simulink model "PreBrakingModel"  (Simulink 8.0)
settings: Solver=ode5  SolverMode=SingleTasking  StartTime=0.0  StopTime=inf  FixedStep=1/1000  RelTol=1e-3
libraries: simulink x27, simulink_extras x2
(part 2 of 2)

== system PreBrakingModel/PreBraking Model/Display module/Display ==
  RPM : Inport
  V : Inport  Port=2
  BrakePressure : Inport  Port=3
  Throttle : Inport  Port=4
  Warning flag 2.6s : Inport  Port=5
  Enable : EnablePort  PropagateVarSize=During execution
  Brake Pressure [bar] : Gain  Gain=100/MaxBrakePressure
  DISPLAY : M-S-Function  FunctionName=msfcn_AEBS_PlotSpeed  Parameters=DisplayFreq DisplaySwitch
  Logical Operator1 : Logic  Operator=OR  Inputs=1  AllPortsSameDT=off  OutDataTypeStr=boolean
  Rounding Function{,1..3} (4 alike) : Rounding  Operator=round  SampleTime=1/DisplayFreq
  wires:
  Rounding Function/1 -> DISPLAY/1
  Rounding Function1/1 -> DISPLAY/2
  Rounding Function2/1 -> DISPLAY/3
  Rounding Function3/1 -> DISPLAY/4
  Brake Pressure [bar]/1 -> Rounding Function2/1
  Logical Operator1/1 -> DISPLAY/5
  RPM/1 -> Rounding Function/1
  V/1 -> Rounding Function1/1
  BrakePressure/1 -> Brake Pressure [bar]/1
  Throttle/1 -> Rounding Function3/1
  Warning flag 2.6s/1 -> Logical Operator1/1

== system PreBrakingModel/PreBraking Model/Interpretation/If Action Subsystem ==
  Action Port : ActionPort  PropagateVarSize=During execution  ActionType=then
  Constant : Constant
  Data Store Write : DataStoreWrite  DataStoreName=full
  wires:
  Constant/1 -> Data Store Write/1

== system PreBrakingModel/PreBraking Model/Interpretation/If Action Subsystem1 ==
  Action Port : ActionPort  PropagateVarSize=During execution  ActionType=then
  Constant : Constant
  Data Store Write : DataStoreWrite  DataStoreName=part
  wires:
  Constant/1 -> Data Store Write/1

== system PreBrakingModel/PreBraking Model/Interpretation/If Action Subsystem2 ==
  Action Port : ActionPort  PropagateVarSize=During execution  ActionType=then
  Constant : Constant  Value=0  SampleTime=min(Tsensor)
  Data Store Write : DataStoreWrite  DataStoreName=part
  wires:
  Constant/1 -> Data Store Write/1

== system PreBrakingModel/PreBraking Model/Radar/Radar ==
  TIS1 Range : Inport
  TIS1 Theta : Inport  Port=2
  TIS2 Range : Inport  Port=3
  TIS2 Theta : Inport  Port=4
  all_flags1.6 : Inport  Port=5
  all_flags2.6 : Inport  Port=6
  all_flags0.6 : Inport  Port=7
  Enable : EnablePort  PropagateVarSize=During execution
  Level-2 M-file S-Function : M-S-Function  FunctionName=msfcn_AEBS_radar_graph  Parameters=RadarFreq TISdet TISMaxRange TISMaxTheta RadarSwitch
  wires:
  TIS1 Range/1 -> Level-2 M-file S-Function/1
  TIS1 Theta/1 -> Level-2 M-file S-Function/2
  TIS2 Range/1 -> Level-2 M-file S-Function/3
  TIS2 Theta/1 -> Level-2 M-file S-Function/4
  all_flags1.6/1 -> Level-2 M-file S-Function/5
  all_flags2.6/1 -> Level-2 M-file S-Function/6
  all_flags0.6/1 -> Level-2 M-file S-Function/7

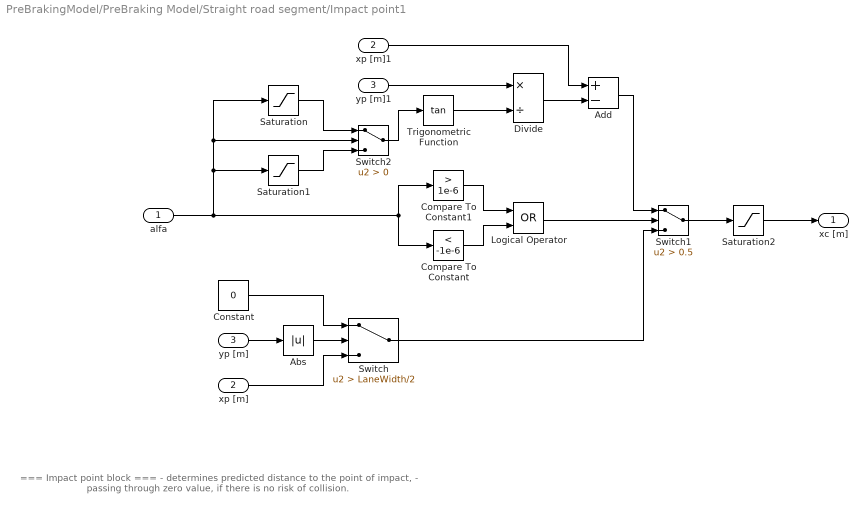
== system PreBrakingModel/PreBraking Model/Straight road segment/Impact point1 ==
  note: === Impact point block ===
      |
      |    - determines predicted distance to the point of impact,
      |    - passing through zero value, if there is no risk of collision.
  alfa : Inport
  xp [m] : Inport  Port=2
  yp [m] : Inport  Port=3
  Abs : Abs
  Add : Sum  Inputs=+-
  Compare To Constant : simulink/Logic and Bit Operations/Compare To Constant  relop=<  const=-1e-6  OutDataTypeStr=uint8  ZeroCross=off
  Compare To Constant1 : simulink/Logic and Bit Operations/Compare To Constant  relop=>  const=1e-6  OutDataTypeStr=uint8  ZeroCross=off
  Constant : Constant  Value=0
  Divide : Product  Inputs=*/
  Logical Operator : Logic  Operator=OR  AllPortsSameDT=off  OutDataTypeStr=boolean
  Saturation : Saturate  UpperLimit=inf  LowerLimit=1e-6
  Saturation1 : Saturate  UpperLimit=-1e-6  LowerLimit=-inf
  Saturation2 : Saturate  UpperLimit=300  LowerLimit=0
  Switch : Switch  Criteria=u2 > Threshold  Threshold=LaneWidth/2
  Switch1 : Switch  Criteria=u2 > Threshold  Threshold=0.5
  Switch2 : Switch  Criteria=u2 > Threshold
  Trigonometric Function : Trigonometry  Operator=tan
  xp [m]1 : InportShadow  Port=2
  yp [m]1 : InportShadow  Port=3
  xc [m] : Outport
  wires:
  yp [m]/1 -> Abs/1
  xp [m]/1 -> Switch/3
  Constant/1 -> Switch/1
  Switch/1 -> Switch1/3
  Abs/1 -> Switch/2
  xp [m]1/1 -> Add/1
  Divide/1 -> Add/2
  yp [m]1/1 -> Divide/1
  Trigonometric Function/1 -> Divide/2
  alfa/1 -> Compare To Constant1/1, Compare To Constant/1, Saturation1/1, Switch2/2, Saturation/1
  Compare To Constant1/1 -> Logical Operator/1
  Compare To Constant/1 -> Logical Operator/2
  Logical Operator/1 -> Switch1/2
  Switch1/1 -> Saturation2/1
  Add/1 -> Switch1/1
  Switch2/1 -> Trigonometric Function/1
  Saturation/1 -> Switch2/1
  Saturation1/1 -> Switch2/3
  Saturation2/1 -> xc [m]/1

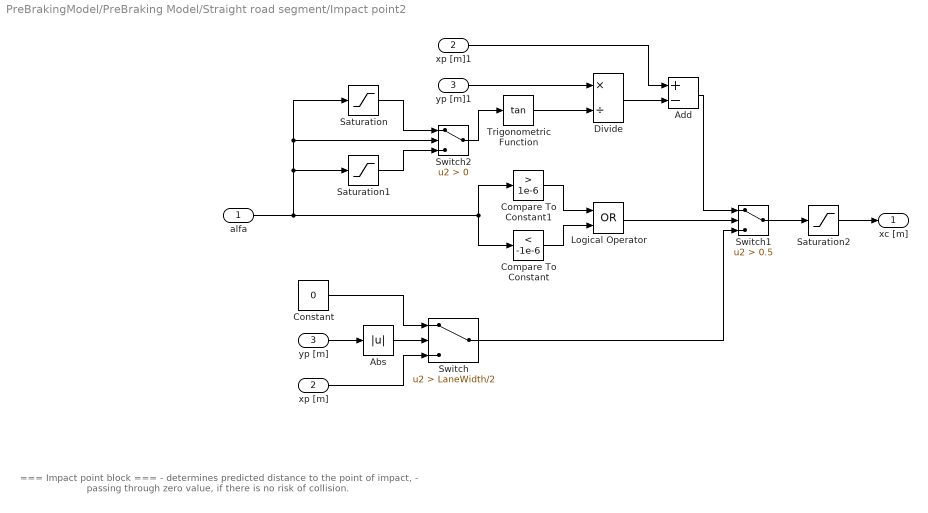
== system PreBrakingModel/PreBraking Model/Straight road segment/Impact point2 ==
  note: === Impact point block ===
      |
      |    - determines predicted distance to the point of impact,
      |    - passing through zero value, if there is no risk of collision.
  alfa : Inport
  xp [m] : Inport  Port=2
  yp [m] : Inport  Port=3
  Abs : Abs
  Add : Sum  Inputs=+-
  Compare To Constant : simulink/Logic and Bit Operations/Compare To Constant  relop=<  const=-1e-6  OutDataTypeStr=uint8  ZeroCross=off
  Compare To Constant1 : simulink/Logic and Bit Operations/Compare To Constant  relop=>  const=1e-6  OutDataTypeStr=uint8  ZeroCross=off
  Constant : Constant  Value=0
  Divide : Product  Inputs=*/
  Logical Operator : Logic  Operator=OR  AllPortsSameDT=off  OutDataTypeStr=boolean
  Saturation : Saturate  UpperLimit=inf  LowerLimit=1e-6
  Saturation1 : Saturate  UpperLimit=-1e-6  LowerLimit=-inf
  Saturation2 : Saturate  UpperLimit=300  LowerLimit=0
  Switch : Switch  Criteria=u2 > Threshold  Threshold=LaneWidth/2
  Switch1 : Switch  Criteria=u2 > Threshold  Threshold=0.5
  Switch2 : Switch  Criteria=u2 > Threshold
  Trigonometric Function : Trigonometry  Operator=tan
  xp [m]1 : InportShadow  Port=2
  yp [m]1 : InportShadow  Port=3
  xc [m] : Outport
  wires:
  yp [m]/1 -> Abs/1
  xp [m]/1 -> Switch/3
  Constant/1 -> Switch/1
  Switch/1 -> Switch1/3
  Abs/1 -> Switch/2
  xp [m]1/1 -> Add/1
  Divide/1 -> Add/2
  yp [m]1/1 -> Divide/1
  Trigonometric Function/1 -> Divide/2
  alfa/1 -> Compare To Constant1/1, Compare To Constant/1, Saturation1/1, Switch2/2, Saturation/1
  Compare To Constant1/1 -> Logical Operator/1
  Compare To Constant/1 -> Logical Operator/2
  Logical Operator/1 -> Switch1/2
  Switch1/1 -> Saturation2/1
  Add/1 -> Switch1/1
  Switch2/1 -> Trigonometric Function/1
  Saturation/1 -> Switch2/1
  Saturation1/1 -> Switch2/3
  Saturation2/1 -> xc [m]/1

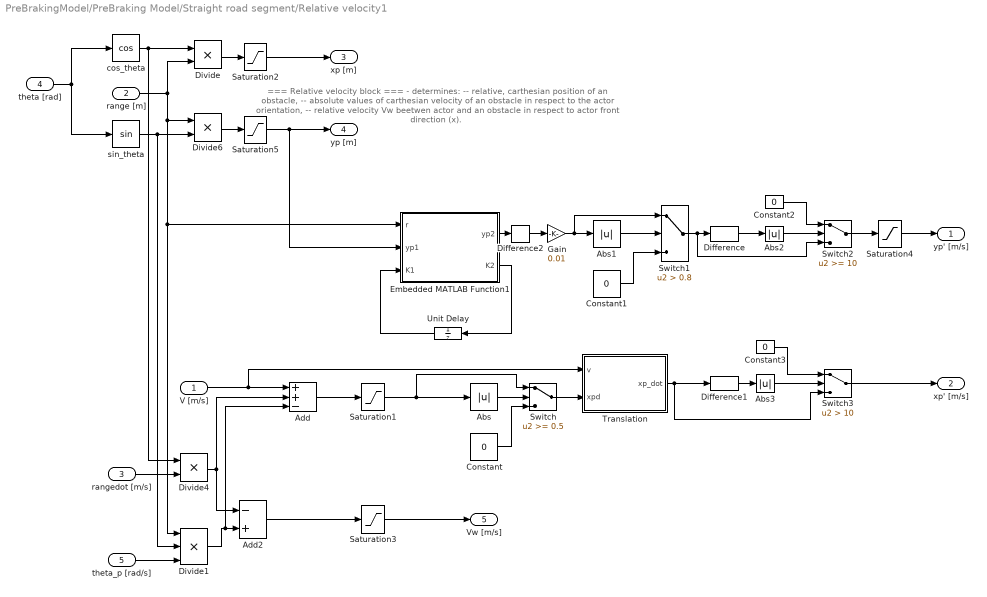
== system PreBrakingModel/PreBraking Model/Straight road segment/Relative velocity1 ==
  note: === Relative velocity block ===
      |
      |    - determines:
      |      -- relative, carthesian position of an obstacle,
      |      -- absolute values of carthesian velocity of an obstacle
      |          in respect to the actor orientation,
      |      -- relative velocity Vw beetwen actor and an obstacle
      |          in respect to actor front direction (x).
  V [m/s] : Inport
  range [m] : Inport  Port=2
  rangedot [m/s] : Inport  Port=3
  theta [rad] : Inport  Port=4
  theta_p [rad/s] : Inport  Port=5
  Abs{,1..3} (4 alike) : Abs
  Add : Sum  Inputs=++-
  Add2 : Sum  Inputs=-+
  Constant{,1..3} (4 alike) : Constant  Value=0
  Difference : simulink/Discrete/Difference  ICPrevInput=zeros(TISdet(1),1)  InputProcessing=Inherited  OutMin=[]  OutMax=[]  OutDataType=fixdt(1, 16)  OutScaling=2^-10  DoSatur=off
  Difference1 : simulink/Discrete/Difference  ICPrevInput=zeros(TISdet(1),1)  InputProcessing=Inherited  OutMin=[]  OutMax=[]  OutDataType=fixdt(1, 16)  OutScaling=2^-10  DoSatur=off
  Difference2 : simulink/Discrete/Difference  ICPrevInput=0.0  InputProcessing=Inherited  OutMin=[]  OutMax=[]  OutDataType=sfix(16)  OutScaling=2^-10  DoSatur=off
  Divide : Product  Inputs=**
  Divide1 : Product  Inputs=***
  Divide4 : Product  Inputs=**
  Divide6 : Product  Inputs=**
  Embedded MATLAB Function1 : MATLAB Function  TreatAsAtomicUnit=on
  Gain : Gain  Gain=0.01
  Saturation1 : Saturate  UpperLimit=50  LowerLimit=-50
  Saturation2 : Saturate  UpperLimit=150  LowerLimit=0
  Saturation3 : Saturate  UpperLimit=50  LowerLimit=-50
  Saturation4 : Saturate  UpperLimit=50  LowerLimit=-50
  Saturation5 : Saturate  UpperLimit=11.8  LowerLimit=-11.8
  Switch : Switch  Threshold=0.5
  Switch1 : Switch  Criteria=u2 > Threshold  Threshold=0.8
  Switch2 : Switch  Threshold=10
  Switch3 : Switch  Criteria=u2 > Threshold  Threshold=10
  Translation : MATLAB Function  TreatAsAtomicUnit=on
  Unit Delay : UnitDelay  InitialCondition=zeros(TISdet(1),50)  SampleTime=-1
  cos_theta : Trigonometry  Operator=cos
  sin_theta : Trigonometry
  yp' [m/s] : Outport
  xp' [m/s] : Outport  Port=2
  xp [m] : Outport  Port=3
  yp [m] : Outport  Port=4
  Vw [m/s] : Outport  Port=5
  wires:
  theta [rad]/1 -> cos_theta/1, sin_theta/1
  Divide/1 -> Saturation2/1
  range [m]/1 -> Divide/2, Divide6/1, Divide1/1, Embedded MATLAB Function1/1(r)
  sin_theta/1 -> Divide6/2, Divide1/2
  cos_theta/1 -> Divide/1, Divide4/1
  Divide6/1 -> Saturation5/1
  theta_p [rad/s]/1 -> Divide1/3
  Add2/1 -> Saturation3/1
  Divide4/1 -> Add2/1, Add/2
  Divide1/1 -> Add2/2, Add/3
  Saturation2/1 -> xp [m]/1
  Saturation5/1 -> Embedded MATLAB Function1/2(yp1), yp [m]/1
  Saturation1/1 -> Abs/1, Switch/1
  V [m/s]/1 -> Translation/1(v), Add/1
  Add/1 -> Saturation1/1
  Abs/1 -> Switch/2
  Constant/1 -> Switch/3
  Switch/1 -> Translation/2(xpd)
  Embedded MATLAB Function1/2(K2) -> Unit Delay/1
  Unit Delay/1 -> Embedded MATLAB Function1/3(K1)
  Embedded MATLAB Function1/1(yp2) -> Difference2/1
  Difference2/1 -> Gain/1
  Abs1/1 -> Switch1/2
  Constant1/1 -> Switch1/3
  Saturation4/1 -> yp' [m/s]/1
  Switch1/1 -> Difference/1, Switch2/3
  Switch2/1 -> Saturation4/1
  Difference/1 -> Abs2/1
  Abs2/1 -> Switch2/2
  Translation/1(xp_dot) -> Switch3/3, Difference1/1
  Abs3/1 -> Switch3/2
  Switch3/1 -> xp' [m/s]/1
  Constant2/1 -> Switch2/1
  Constant3/1 -> Switch3/1
  Difference1/1 -> Abs3/1
  rangedot [m/s]/1 -> Divide4/2
  Gain/1 -> Abs1/1, Switch1/1
  Saturation3/1 -> Vw [m/s]/1

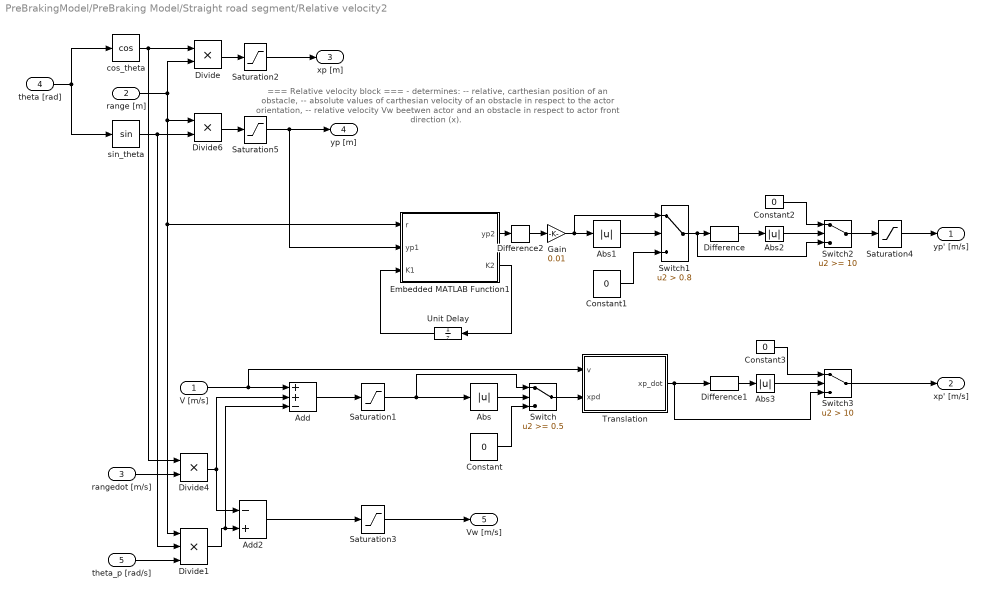
== system PreBrakingModel/PreBraking Model/Straight road segment/Relative velocity2 ==
  note: === Relative velocity block ===
      |
      |    - determines:
      |      -- relative, carthesian position of an obstacle,
      |      -- absolute values of carthesian velocity of an obstacle
      |          in respect to the actor orientation,
      |      -- relative velocity Vw beetwen actor and an obstacle
      |          in respect to actor front direction (x).
  V [m/s] : Inport
  range [m] : Inport  Port=2
  rangedot [m/s] : Inport  Port=3
  theta [rad] : Inport  Port=4
  theta_p [rad/s] : Inport  Port=5
  Abs{,1..3} (4 alike) : Abs
  Add : Sum  Inputs=++-
  Add2 : Sum  Inputs=-+
  Constant{,1..3} (4 alike) : Constant  Value=0
  Difference : simulink/Discrete/Difference  ICPrevInput=zeros(TISdet(2),1)  InputProcessing=Inherited  OutMin=[]  OutMax=[]  OutDataType=fixdt(1, 16)  OutScaling=2^-10  DoSatur=off
  Difference1 : simulink/Discrete/Difference  ICPrevInput=zeros(TISdet(2),1)  InputProcessing=Inherited  OutMin=[]  OutMax=[]  OutDataType=fixdt(1, 16)  OutScaling=2^-10  DoSatur=off
  Difference2 : simulink/Discrete/Difference  ICPrevInput=0.0  InputProcessing=Inherited  OutMin=[]  OutMax=[]  OutDataType=sfix(16)  OutScaling=2^-10  DoSatur=off
  Divide : Product  Inputs=**
  Divide1 : Product  Inputs=***
  Divide4 : Product  Inputs=**
  Divide6 : Product  Inputs=**
  Embedded MATLAB Function1 : MATLAB Function  TreatAsAtomicUnit=on  SystemSampleTime=0.01
  Gain : Gain  Gain=0.01
  Saturation1 : Saturate  UpperLimit=50  LowerLimit=-50
  Saturation2 : Saturate  UpperLimit=150  LowerLimit=0
  Saturation3 : Saturate  UpperLimit=50  LowerLimit=-50
  Saturation4 : Saturate  UpperLimit=50  LowerLimit=-50
  Saturation5 : Saturate  UpperLimit=11.8  LowerLimit=-11.8
  Switch : Switch  Threshold=0.5
  Switch1 : Switch  Criteria=u2 > Threshold  Threshold=0.8
  Switch2 : Switch  Threshold=10
  Switch3 : Switch  Criteria=u2 > Threshold  Threshold=10
  Translation : MATLAB Function  TreatAsAtomicUnit=on
  Unit Delay : UnitDelay  InitialCondition=zeros(TISdet(2),50)  SampleTime=-1
  cos_theta : Trigonometry  Operator=cos
  sin_theta : Trigonometry
  yp' [m/s] : Outport
  xp' [m/s] : Outport  Port=2
  xp [m] : Outport  Port=3
  yp [m] : Outport  Port=4
  Vw [m/s] : Outport  Port=5
  wires:
  rangedot [m/s]/1 -> Divide4/2
  Difference1/1 -> Abs3/1
  Constant3/1 -> Switch3/1
  Constant2/1 -> Switch2/1
  Switch3/1 -> xp' [m/s]/1
  Abs3/1 -> Switch3/2
  Translation/1(xp_dot) -> Difference1/1, Switch3/3
  Abs2/1 -> Switch2/2
  Difference/1 -> Abs2/1
  Switch2/1 -> Saturation4/1
  Switch1/1 -> Switch2/3, Difference/1
  Saturation4/1 -> yp' [m/s]/1
  Constant1/1 -> Switch1/3
  Abs1/1 -> Switch1/2
  Gain/1 -> Switch1/1, Abs1/1
  Embedded MATLAB Function1/1(yp2) -> Difference2/1
  Unit Delay/1 -> Embedded MATLAB Function1/3(K1)
  Embedded MATLAB Function1/2(K2) -> Unit Delay/1
  Switch/1 -> Translation/2(xpd)
  Constant/1 -> Switch/3
  Abs/1 -> Switch/2
  Add/1 -> Saturation1/1
  V [m/s]/1 -> Translation/1(v), Add/1
  Saturation1/1 -> Switch/1, Abs/1
  Saturation5/1 -> yp [m]/1, Embedded MATLAB Function1/2(yp1)
  Saturation2/1 -> xp [m]/1
  Divide1/1 -> Add/3, Add2/2
  Divide4/1 -> Add/2, Add2/1
  Add2/1 -> Saturation3/1
  theta_p [rad/s]/1 -> Divide1/3
  Divide6/1 -> Saturation5/1
  cos_theta/1 -> Divide/1, Divide4/1
  sin_theta/1 -> Divide6/2, Divide1/2
  range [m]/1 -> Embedded MATLAB Function1/1(r), Divide1/1, Divide6/1, Divide/2
  Divide/1 -> Saturation2/1
  theta [rad]/1 -> cos_theta/1, sin_theta/1
  Difference2/1 -> Gain/1
  Saturation3/1 -> Vw [m/s]/1

== system PreBrakingModel/PreBraking Model/Straight road segment/T0.6 ==
  note: === T1.6 block ==
      |
      |    - compare TTC and output adequate binary flag.
  TTC : Inport
  Constant TTC : Inport  Port=2
  Gain : Gain  Gain=2
  Gain2 : Gain  Gain=ones(TISdet(2),1)
  Relational Operator1 : RelationalOperator  Operator=<  OutDataTypeStr=fixdt(1,16)
  Switch : Switch  Criteria=u2 > Threshold
  all_flags_0,6 : Outport
  wires:
  Switch/1 -> Relational Operator1/1
  TTC/1 -> Switch/2, Switch/1
  Constant TTC/1 -> Gain2/1
  Gain/1 -> Switch/3
  Gain2/1 -> Gain/1, Relational Operator1/2
  Relational Operator1/1 -> all_flags_0,6/1

== system PreBrakingModel/PreBraking Model/Straight road segment/T1.6 ==
  note: === T1.6 block ==
      |
      |    - compare TTC and output adequate binary flag.
  TTC : Inport
  Constant TTC : Inport  Port=2
  Gain : Gain  Gain=2
  Gain2 : Gain  Gain=ones(TISdet(1),1)
  Relational Operator1 : RelationalOperator  Operator=<  OutDataTypeStr=fixdt(1,16)
  Switch : Switch  Criteria=u2 > Threshold
  median filter : Subsystem
  all_flags_1.6 : Outport
  wires:
  Switch/1 -> Relational Operator1/1
  Relational Operator1/1 -> median filter/1(Flag in)
  TTC/1 -> Switch/2, Switch/1
  Constant TTC/1 -> Gain2/1
  Gain/1 -> Switch/3
  Gain2/1 -> Gain/1, Relational Operator1/2
  median filter/1(Flag out) -> all_flags_1.6/1

== system PreBrakingModel/PreBraking Model/Straight road segment/T2.6 ==
  note: === T1.6 block ==
      |
      |    - compare TTC and output adequate binary flag.
  TTC : Inport
  Constant TTC : Inport  Port=2
  Gain : Gain  Gain=2
  Gain2 : Gain  Gain=ones(TISdet(1),1)
  Relational Operator1 : RelationalOperator  Operator=<  OutDataTypeStr=fixdt(1,16)
  Switch : Switch  Criteria=u2 > Threshold
  median filter : Subsystem
  all_flags_2.6 : Outport
  wires:
  Switch/1 -> Relational Operator1/1
  TTC/1 -> Switch/2, Switch/1
  Constant TTC/1 -> Gain2/1
  Gain/1 -> Switch/3
  Gain2/1 -> Gain/1, Relational Operator1/2
  Relational Operator1/1 -> median filter/1(Flag in)
  median filter/1(Flag out) -> all_flags_2.6/1

== system PreBrakingModel/PreBraking Model/Straight road segment/THETA Derivative1 ==
  note: === Theta derivative block ===
      |
      |    - computs derivative of the theta using linear
      |       extrapolation and correction method
  range [m] : Inport
  theta [rad] : Inport  Port=2
  Abs1 : Abs
  Deriv correction : MATLAB Function  TreatAsAtomicUnit=on
  Difference1 : simulink/Discrete/Difference  ICPrevInput=0.0  InputProcessing=Inherited  OutMin=[]  OutMax=[]  OutDataType=sfix(16)  OutScaling=2^-10  DoSatur=off
  Difference2 : simulink/Discrete/Difference  ICPrevInput=0.0  InputProcessing=Inherited  OutMin=[]  OutMax=[]  OutDataType=sfix(16)  OutScaling=2^-10  DoSatur=off
  Digital Clock : DigitalClock  SampleTime=min(Tsensor)
  Gain : Gain  Gain=Tsensor(2)
  Gain1 : Gain  Gain=Tsensor(2)
  Switch : Switch  Threshold=2
  Theta extrapolation : MATLAB Function  TreatAsAtomicUnit=on
  Unit Delay : UnitDelay  InitialCondition=zeros(TISdet(2),1)  SampleTime=-1
  Unit Delay1 : UnitDelay  InitialCondition=zeros(TISdet(2),10,2)  SampleTime=-1
  Unit Delay2 : UnitDelay  InitialCondition=zeros(TISdet(2),1)  SampleTime=-1
  theta_dot [rad/s] : Outport
  wires:
  Unit Delay2/1 -> Deriv correction/2(thp)
  Gain1/1 -> Deriv correction/3(thd)
  Theta extrapolation/1(th2) -> Deriv correction/1(th), Unit Delay2/1, Difference1/1
  range [m]/1 -> Theta extrapolation/1(r)
  Gain/1 -> Theta extrapolation/3(thd)
  Digital Clock/1 -> Theta extrapolation/4(time)
  Unit Delay1/1 -> Theta extrapolation/5(K1)
  Theta extrapolation/2(K2) -> Unit Delay1/1
  theta [rad]/1 -> Theta extrapolation/2(th1), Difference2/1
  Deriv correction/1(th_dot) -> Switch/3, Abs1/1
  Switch/1 -> theta_dot [rad/s]/1, Unit Delay/1
  Abs1/1 -> Switch/2
  Unit Delay/1 -> Switch/1
  Difference2/1 -> Gain/1
  Difference1/1 -> Gain1/1

== system PreBrakingModel/PreBraking Model/Straight road segment/THETA Derivative2 ==
  note: === Theta derivative block ===
      |
      |    - computs derivative of the theta using linear
      |       extrapolation and correction method
  range [m] : Inport
  theta [rad] : Inport  Port=2
  Abs1 : Abs
  Deriv correction : MATLAB Function  TreatAsAtomicUnit=on
  Difference1 : simulink/Discrete/Difference  ICPrevInput=0.0  InputProcessing=Inherited  OutMin=[]  OutMax=[]  OutDataType=sfix(16)  OutScaling=2^-10  DoSatur=off
  Difference2 : simulink/Discrete/Difference  ICPrevInput=0.0  InputProcessing=Inherited  OutMin=[]  OutMax=[]  OutDataType=sfix(16)  OutScaling=2^-10  DoSatur=off
  Digital Clock : DigitalClock  SampleTime=min(Tsensor)
  Gain : Gain  Gain=Tsensor(1)
  Gain1 : Gain  Gain=Tsensor(1)
  Switch : Switch  Threshold=2
  Theta extrapolation : MATLAB Function  TreatAsAtomicUnit=on
  Unit Delay : UnitDelay  InitialCondition=zeros(TISdet(1),1)  SampleTime=-1
  Unit Delay1 : UnitDelay  InitialCondition=zeros(TISdet(1),10,2)  SampleTime=-1
  Unit Delay2 : UnitDelay  InitialCondition=zeros(TISdet(1),1)  SampleTime=-1
  theta_dot [rad/s] : Outport
  wires:
  Unit Delay2/1 -> Deriv correction/2(thp)
  Gain1/1 -> Deriv correction/3(thd)
  Theta extrapolation/1(th2) -> Deriv correction/1(th), Unit Delay2/1, Difference1/1
  range [m]/1 -> Theta extrapolation/1(r)
  Gain/1 -> Theta extrapolation/3(thd)
  Digital Clock/1 -> Theta extrapolation/4(time)
  Unit Delay1/1 -> Theta extrapolation/5(K1)
  Theta extrapolation/2(K2) -> Unit Delay1/1
  theta [rad]/1 -> Theta extrapolation/2(th1), Difference2/1
  Deriv correction/1(th_dot) -> Switch/3, Abs1/1
  Switch/1 -> theta_dot [rad/s]/1, Unit Delay/1
  Abs1/1 -> Switch/2
  Unit Delay/1 -> Switch/1
  Difference2/1 -> Gain/1
  Difference1/1 -> Gain1/1

== system PreBrakingModel/PreBraking Model/Straight road segment/TTC computing ==
  xc [m] : Inport
  Vw [m/s] : Inport  Port=2
  Compare To Constant : simulink/Logic and Bit Operations/Compare To Constant  relop===  const=1e-6  OutDataTypeStr=uint8  ZeroCross=off
  Constant : Constant  Value=0
  Data Type Conversion : DataTypeConversion
  Divide : Product  Inputs=/*
  Saturation : Saturate  UpperLimit=inf  LowerLimit=1e-6
  Switch : Switch  Criteria=u2 > Threshold
  Switch1 : Switch  Criteria=u2 > Threshold  Threshold=0.5
  TTC : Outport  InitialOutput=0
  wires:
  Vw [m/s]/1 -> Switch/2, Switch/1
  Constant/1 -> Switch1/1, Switch/3
  Switch/1 -> Saturation/1
  Saturation/1 -> Divide/1, Compare To Constant/1
  Compare To Constant/1 -> Data Type Conversion/1
  xc [m]/1 -> Divide/2
  Divide/1 -> Switch1/3
  Switch1/1 -> TTC/1
  Data Type Conversion/1 -> Switch1/2

== system PreBrakingModel/PreBraking Model/Straight road segment/TTC computing1 ==
  xc [m] : Inport
  Vw [m/s] : Inport  Port=2
  Compare To Constant : simulink/Logic and Bit Operations/Compare To Constant  relop===  const=1e-6  OutDataTypeStr=uint8  ZeroCross=off
  Constant : Constant  Value=0
  Data Type Conversion : DataTypeConversion
  Divide : Product  Inputs=/*
  Saturation : Saturate  UpperLimit=inf  LowerLimit=1e-6
  Switch : Switch  Criteria=u2 > Threshold
  Switch1 : Switch  Criteria=u2 > Threshold  Threshold=0.5
  TTC : Outport  InitialOutput=0
  wires:
  Vw [m/s]/1 -> Switch/2, Switch/1
  Constant/1 -> Switch/3, Switch1/1
  Switch/1 -> Saturation/1
  Saturation/1 -> Divide/1, Compare To Constant/1
  Compare To Constant/1 -> Data Type Conversion/1
  xc [m]/1 -> Divide/2
  Divide/1 -> Switch1/3
  Switch1/1 -> TTC/1
  Data Type Conversion/1 -> Switch1/2

== system PreBrakingModel/PreBraking Model/Straight road segment/alfa ==
  yp'1 : Inport
  xp' : Inport  Port=2
  Abs : Abs
  Compare To Constant : simulink/Logic and Bit Operations/Compare To Constant  relop===  const=pi/2  OutDataTypeStr=uint8
  Constant : Constant  Value=0
  Switch : Switch  Criteria=u2 > Threshold
  four quadrant atan : Trigonometry  Operator=atan2
  alfa1 : Outport
  wires:
  yp'1/1 -> four quadrant atan/1
  xp'/1 -> four quadrant atan/2
  four quadrant atan/1 -> Abs/1, Switch/3
  Abs/1 -> Compare To Constant/1
  Compare To Constant/1 -> Switch/2
  Constant/1 -> Switch/1
  Switch/1 -> alfa1/1

== system PreBrakingModel/PreBraking Model/Straight road segment/alfa1 ==
  yp'1 : Inport
  xp' : Inport  Port=2
  Abs : Abs
  Compare To Constant : simulink/Logic and Bit Operations/Compare To Constant  relop===  const=pi/2  OutDataTypeStr=uint8
  Constant : Constant  Value=0
  Switch : Switch  Criteria=u2 > Threshold
  four quadrant atan : Trigonometry  Operator=atan2
  alfa1 : Outport
  wires:
  yp'1/1 -> four quadrant atan/1
  xp'/1 -> four quadrant atan/2
  four quadrant atan/1 -> Abs/1, Switch/3
  Abs/1 -> Compare To Constant/1
  Compare To Constant/1 -> Switch/2
  Constant/1 -> Switch/1
  Switch/1 -> alfa1/1

== system PreBrakingModel/PreBraking Model/Bend road segment/T1.6/median filter ==
  Flag in : Inport
  Memory : Memory  InheritSampleTime=on
  Memory1 : Memory  InheritSampleTime=on
  Mux : Mux  Inputs=3
  median function : MATLAB Function  TreatAsAtomicUnit=on
  Flag out : Outport
  wires:
  Flag in/1 -> Mux/1, Memory/1
  Memory/1 -> Mux/2, Memory1/1
  Memory1/1 -> Mux/3
  Mux/1 -> median function/1(u)
  median function/1(y) -> Flag out/1

== system PreBrakingModel/PreBraking Model/Bend road segment/T2.6/median filter ==
  Flag in : Inport
  Memory : Memory  InheritSampleTime=on
  Memory1 : Memory  InheritSampleTime=on
  Mux : Mux  Inputs=3
  median function : MATLAB Function  TreatAsAtomicUnit=on
  Flag out : Outport
  wires:
  Flag in/1 -> Mux/1, Memory/1
  Memory/1 -> Mux/2, Memory1/1
  Memory1/1 -> Mux/3
  Mux/1 -> median function/1(u)
  median function/1(y) -> Flag out/1

== system PreBrakingModel/PreBraking Model/Straight road segment/T1.6/median filter ==
  Flag in : Inport
  Memory : Memory  InheritSampleTime=on
  Memory1 : Memory  InheritSampleTime=on
  Mux : Mux  Inputs=3
  median function : MATLAB Function  TreatAsAtomicUnit=on
  Flag out : Outport
  wires:
  Flag in/1 -> Mux/1, Memory/1
  Memory/1 -> Mux/2, Memory1/1
  Memory1/1 -> Mux/3
  Mux/1 -> median function/1(u)
  median function/1(y) -> Flag out/1

== system PreBrakingModel/PreBraking Model/Straight road segment/T2.6/median filter ==
  Flag in : Inport
  Memory : Memory  InheritSampleTime=on
  Memory1 : Memory  InheritSampleTime=on
  Mux : Mux  Inputs=3
  median function : MATLAB Function  TreatAsAtomicUnit=on
  Flag out : Outport
  wires:
  Flag in/1 -> Mux/1, Memory/1
  Memory/1 -> Mux/2, Memory1/1
  Memory1/1 -> Mux/3
  Mux/1 -> median function/1(u)
  median function/1(y) -> Flag out/1

== matlab function PreBraking Model/Straight road segment/Relative velocity2/Embedded MATLAB Function1 ==
  data: r input double; yp2 output double; yp1 input double; K1 input double; K2 output double; TISdet parameter double; TISMaxRange parameter double
function [yp2, K2] = modif(r, yp1, K1, TISdet, TISMaxRange)
%#codegen
% Interpolating yp value.

K2 = K1;
yp2 = yp1;

d = 50;

% Adding point
for i = 1 : TISdet(2)
   if r(i) ~= 5*TISMaxRange(2) 
      K2(i,1:d-1) = K2(i,2:d);
      K2(i,d) = yp1(i);
   end
end

% Choosing what to take
for i = 1 : TISdet(2)
    s = 0;
    suma = 0;
    for j = 1 : 50
        if K2(i,j) ~= 0
            suma = suma + K2(i,j);
            s = s + 1;
        end
    end
    yp2(i) = suma/s;
end

% Returning, if object is not detected
for i = 1: TISdet(2)
    if r(i) == 30 && yp1(i) == 0
        K2(i,:,:) = zeros(d,1);
        yp2(i) = 0;
    end    
end

== matlab function PreBraking Model/Straight road segment/Relative velocity2/Translation ==
  data: v input double; xpd input double; xp_dot output double; TISdet parameter double
function xp_dot = trans(v, xpd, TISdet)
%#codegen
%Translation of the value

xp_dot = xpd;
for i = 1 : TISdet(2)
    if xpd(i) == v
        xp_dot(i) =0;
    end
end
end

== matlab function PreBraking Model/TIS2sorting_fun/Embedded MATLAB Function ==
  data: range input double; indx input double; RANGE output double; TISdet parameter double
function RANGE = dis(range, indx, TISdet)
%#codegen

RANGE = zeros(TISdet(2),1);
for i = 1 : length(indx)
    if indx(i) ~= 0
        RANGE(i) = range(indx(i));
    else
        RANGE(i) = 0;
    end
end

== matlab function PreBraking Model/TIS2sorting_fun/Embedded MATLAB Function1 ==
  data: indx input double; THETA output double; theta input double; TISdet parameter double
function THETA = ang(indx, theta, TISdet)
%#codegen

THETA = zeros(TISdet(2),1);
for i = 1 : length(indx)
    if indx(i) ~= 0
        THETA(i) = theta(indx(i));
    else
        THETA(i) = 0;
    end
end

== matlab function PreBraking Model/TIS2sorting_fun/Embedded MATLAB Function2 ==
  data: indx input double; RANGEDOT output double; rangedot input double; TISdet parameter double
function RANGEDOT = vel(indx, rangedot, TISdet)
%#codegen

RANGEDOT = zeros(TISdet(2),1);
for i = 1 : length(indx)
    if indx(i) ~= 0
        RANGEDOT(i) = rangedot(indx(i));
    else
        RANGEDOT(i) = 0;
    end
end

== matlab function PreBraking Model/TIS1sorting_fun/Embedded MATLAB Function ==
  data: range input double; indx input double; RANGE output double; TISdet parameter double
function RANGE = dis(range, indx, TISdet)
%#codegen

RANGE = zeros(TISdet(1),1);
for i = 1 : length(indx)
    if indx(i) ~= 0
        RANGE(i) = range(indx(i));
    else
        RANGE(i) = 0;
    end
end

== matlab function PreBraking Model/Straight road segment/Relative velocity1/Translation ==
  data: v input double; xpd input double; xp_dot output double; TISdet parameter double
function xp_dot = trans(v, xpd, TISdet)
%#codegen
%Translation of the value

xp_dot = xpd;
for i = 1 : TISdet(1)
    if xpd(i) == v
        xp_dot(i) = 0;
    end
end
end

== matlab function PreBraking Model/Straight road segment/Relative velocity1/Embedded MATLAB Function1 ==
  settings: updateMethod=DISCRETE
  data: r input double; yp2 output double; yp1 input double; K1 input double; K2 output double; TISdet parameter double; TISMaxRange parameter double
function [yp2, K2] = modif(r, yp1, K1, TISdet, TISMaxRange)
%#codegen
% Interpolating yp value.

K2 = K1;
yp2 = yp1;

d = 50;

% Adding point
for i = 1 : TISdet(1)
   if r(i) ~= TISMaxRange(1)
      K2(i,1:d-1) = K2(i,2:d);
      K2(i,d) = yp1(i);
   end
end

% Choosing what to take
for i = 1 : TISdet(1)
    s = 0;
    suma = 0;
    for j = 1 : 50
        if K2(i,j) ~= 0
            suma = suma + K2(i,j);
            s = s + 1;
        end
    end
    yp2(i) = suma/s;
end

% Returning, if object is not detected
for i = 1: TISdet(1)
    if r(i) == TISMaxRange(1) && yp1(i) == 0
        K2(i,:,:) = zeros(d,1);
        yp2(i) = 0;
    end    
end

== matlab function PreBraking Model/TIS1sorting_fun/Embedded MATLAB Function1 ==
  data: indx input double; THETA output double; theta input double; TISdet parameter double
function THETA = ang(indx, theta, TISdet)
%#codegen

THETA = zeros(TISdet(1),1);
for i = 1 : length(indx)
    if indx(i) ~= 0
        THETA(i) = theta(indx(i));
    else
        THETA(i) = 0;
    end
end

== matlab function PreBraking Model/TIS1sorting_fun/Embedded MATLAB Function2 ==
  data: indx input double; RANGEDOT output double; rangedot input double; TISdet parameter double
function RANGEDOT = vel(indx, rangedot, TISdet)
%#codegen

RANGEDOT = zeros(TISdet(1),1);
for i = 1 : length(indx)
    if indx(i) ~= 0
        RANGEDOT(i) = rangedot(indx(i));
    else
        RANGEDOT(i) = 0;
    end
end

== matlab function PreBraking Model/TIS1sorting_fun/MATLAB Function ==
  data: indxp input double; indx output double; range input double; TISdet parameter double
function indx = sorts(indxp, range, TISdet)
%#codegen

size = TISdet(1);

indx = indxp;

for i = 1 : size
    if ( indx(i) ~= 0 ) && ( range(i) == 0)
        indx(i) = 0;
    end
end

for i = 1 : size
    if indx(i) ~= 0
        range(i) = 0;
    end
end

for i = 1 : size
    if range(i) ~= 0
       j = 1;
       while( indx(j) )
           j = j + 1;
       end
       if j ~= size
           indx(j) = i;
       end
    end
end
indx = round(indx);
end

== matlab function PreBraking Model/TIS2sorting_fun/MATLAB Function ==
  data: indxp input double; indx output double; range input double; TISdet parameter double
function indx = sorts(indxp, range, TISdet)
%#codegen

size = TISdet(2);

indx = indxp;

for i = 1 : size
    if ( indx(i) ~= 0 ) && ( range(i) == 0)
        indx(i) = 0;
    end
end

for i = 1 : size
    if indx(i) ~= 0
        range(i) = 0;
    end
end

for i = 1 : size
    if range(i) ~= 0
       j = 1;
       while( indx(j) )
           j = j + 1;
       end
       if j ~= size
           indx(j) = i;
       end
    end
end
indx = round(indx);
end

== matlab function PreBraking Model/Straight road segment/THETA Derivative1/Deriv correction ==
  data: th input double; thp input double; thd input double; th_dot output double; TISdet parameter double
function th_dot = stopping(th, thp, thd, TISdet)
%#codegen
% Stopping if nothing is detected.

th_dot = thd;
for i = 1 : TISdet(2)
    if (th(i)==0 && thp(i)~=0) || (th(i)~=0 && thp(i)==0)
        th_dot(i) = 0;
    end
end
end

== matlab function PreBraking Model/Straight road segment/THETA Derivative2/Deriv correction ==
  data: th input double; thp input double; thd input double; th_dot output double; TISdet parameter double
function th_dot = stopping(th, thp, thd, TISdet)
%#codegen
% Stopping if nothing is detected.

th_dot = thd;
for i = 1 : TISdet(1)
    if (th(i)==0 && thp(i)~=0) || (th(i)~=0 && thp(i)==0)
        th_dot(i) = 0;
    end
end
end

== matlab function PreBraking Model/Straight road segment/THETA Derivative2/Theta extrapolation ==
  data: r input double; th1 input double; th2 output double; thd input double; time input double; K1 input double; K2 output double; TISdet parameter double; TISMaxRange parameter double
function [th2, K2] = modif(r, th1, thd, time, K1, TISdet, TISMaxRange)
%#codegen
% Interpolating theta value.

K2 = K1;
th2 = th1;

d = 10;

% Finding points used in interpolation/extrapolation.
for i = 1 : TISdet(1)
    if thd(i) ~= 0
        K2(i,1:d-1,:) = K2(i,2:d,:);
        K2(i,  d,1) = time;
        K2(i,  d,2) = th1(i);
    end
end

% Extrapolation
for i = 1 : TISdet(1)
    j = 1;
    while j < d+1 && K2(i,j,1) == 0
        j = j + 1;
    end
    
    if j > d-2
        th2(i) = th1(i);
    else
        th2(i) = interp1(K2(i,d-2:d,1),K2(i,d-2:d,2),time,'linear','extrap');
    end
end

% Returning, if object is not detected
for i = 1: TISdet(1)
    if r(i) == TISMaxRange(1) && th1(i) == 0
        K2(i,:,:) = zeros(d,2);
        th2(i) = 0;
    end    
end

end

== matlab function PreBraking Model/Straight road segment/THETA Derivative1/Theta extrapolation ==
  data: r input double; th1 input double; th2 output double; thd input double; time input double; K1 input double; K2 output double; TISdet parameter double; TISMaxRange parameter double
function [th2, K2] = modif(r, th1, thd, time, K1, TISdet, TISMaxRange)
%#codegen
% Interpolating theta value.

K2 = K1;
th2 = th1;

d = 10;

% Finding points used in interpolation/extrapolation.
for i = 1 : TISdet(2)
    if thd(i) ~= 0
        K2(i,1:d-1,:) = K2(i,2:d,:);
        K2(i,  d,1) = time;
        K2(i,  d,2) = th1(i);
    end
end

% Extrapolation
for i = 1 : TISdet(2)
    j = 1;
    while j < d+1 && K2(i,j,1) == 0
        j = j + 1;
    end
    
    if j > d-2
        th2(i) = th1(i);
    else
        th2(i) = interp1(K2(i,d-2:d,1),K2(i,d-2:d,2),time,'linear','extrap');
    end
end

% Returning, if object is not detected
for i = 1: TISdet(2)
    if r(i) == 5*TISMaxRange(2) && th1(i) == 0
        K2(i,:,:) = zeros(d,2);
        th2(i) = 0;
    end    
end

end

== matlab function PreBraking Model/Bend road segment/T2.6/median filter/median function ==
  data: u input double; y output double; TISdet parameter double
function y = fcn(u, TISdet)
%#codegen


nr = 1;
y = zeros(TISdet(nr),1,'int16');

for kk = 1 : TISdet(nr)
    z = 0;
    w = 0;
    for ii = 0 : 2
        if u(TISdet(nr)*ii+kk) == true
            w = w + 1;
        else
            z = z + 1;
        end
    end
    
    if w > z
        y(kk) = int16(1);
    end
end

end

== matlab function PreBraking Model/Bend road segment/T1.6/median filter/median function ==
  data: u input double; y output double; TISdet parameter double
function y = fcn(u, TISdet)
%#codegen


nr = 1;
y = zeros(TISdet(nr),1,'int16');

for kk = 1 : TISdet(nr)
    z = 0;
    w = 0;
    for ii = 0 : 2
        if u(TISdet(nr)*ii+kk) == true
            w = w + 1;
        else
            z = z + 1;
        end
    end
    
    if w > z
        y(kk) = int16(1);
    end
end

end

== matlab function PreBraking Model/Straight road segment/T1.6/median filter/median function ==
  data: u input double; y output double; TISdet parameter double
function y = fcn(u, TISdet)
%#codegen


nr = 1;
y = zeros(TISdet(nr),1,'int16');

for kk = 1 : TISdet(nr)
    z = 0;
    w = 0;
    for ii = 0 : 2
        if u(TISdet(nr)*ii+kk) == true
            w = w + 1;
        else
            z = z + 1;
        end
    end
    
    if w > z
        y(kk) = int16(1);
    end
end

end

== matlab function PreBraking Model/Straight road segment/T2.6/median filter/median function ==
  data: u input double; y output double; TISdet parameter double
function y = fcn(u, TISdet)
%#codegen


nr = 1;
y = zeros(TISdet(nr),1,'int16');

for kk = 1 : TISdet(nr)
    z = 0;
    w = 0;
    for ii = 0 : 2
        if u(TISdet(nr)*ii+kk) == true
            w = w + 1;
        else
            z = z + 1;
        end
    end
    
    if w > z
        y(kk) = int16(1);
    end
end

end
